simulink model "sm_aerial_trajectory"  (R2020b)
settings: Solver=ode45  StartTime=0.0  StopTime=2*T_gait-T_stance  MaxStep=0.001  RelTol=1e-3  EnableMultiTasking=on
InitFcn:
  | if (~exist('T_gait') || ~exist('T_stance'))
  |   sm_robot_run_4legs_param_def_load(bdroot)
  | end
values from neighbouring files (symbols this model uses):
  accel_aerial = (-leg_angle0-(T_gait-T_stance/2)*leg_vel0)/(0.5*(T_gait-T_stance/2)^2)    [kinematic_walking.m]
  T_gait = leg_angle.time(end)    [kinematic_walking.m]
  T_stance = 2*stance.time(idx_stance)    [kinematic_walking.m]
undefined symbols (not defined in the file or in its folder): leg_angle0, leg_vel0
CloseFcn:
  | try,close(h1_sm_robot_run_02_aerial_trajectory),end
  | clear h1_sm_robot_run_02_aerial_trajectory
  | 
  | clear logsout_sm_robot_run_02_aerial_trajectory
Description:
  | Copyright 2012-2020 The MathWorks, Inc.
settings Model: Creator=rhyde  LastModifiedBy=tedsa
settings DataIOCC: SaveFormat=Array  ReturnWorkspaceOutputs=off  SignalLoggingName=logsout_sm_robot_run_02_aerial_trajectory
settings OptimizationCC: ExpressionDepthLimit=2147483647  InitFltsAndDblsToZero=on  LifeSpan=inf
settings DebuggingCC: UnderspecifiedInitializationDetection=Classic  MergeDetectMultiDrivingBlocksExec=none  SolverPrmCheckMsg=warning  FcnCallInpInsideContextMsg=warning  StateNameClashWarn=warning  PregeneratedLibrarySubsystemCodeDiagnostic=none  SFUnexpectedBacktrackingDiag=warning  SFNoUnconditionalDefaultTransitionDiag=warning  SFExecutionAtInitializationDiag=none  ArithmeticOperatorsInVariantConditions=warning
settings HardwareCC: ProdBitPerPointer=32  ProdBitPerSizeT=32  ProdBitPerPtrDiffT=32  ProdLargestAtomicFloat=None  ProdIntDivRoundTo=Undefined  ProdEndianess=Unspecified  ProdWordSize=32  ProdHWDeviceType=32-bit Generic
settings ModelReferenceCC: PropagateSignalLabelsOutOfModel=off
settings SFSimCC: SimUseLocalCustomCode=off  CustomCodeUndefinedFunction=UseInterfaceOnly
settings RTWCC: RTWUseLocalCustomCode=off
settings CodeAppCC: StateflowObjectComments=on
settings GRTTargetCC: TargetLangStandard=C89/C90 (ANSI)  CombineOutputUpdateFcns=off  GRTInterface=on
settings ConfigComp: CovMetricSettings=dw  CovSaveCumulativeToWorkspaceVar=on  CovSaveSingleToWorkspaceVar=on  CovExternalEMLEnable=off

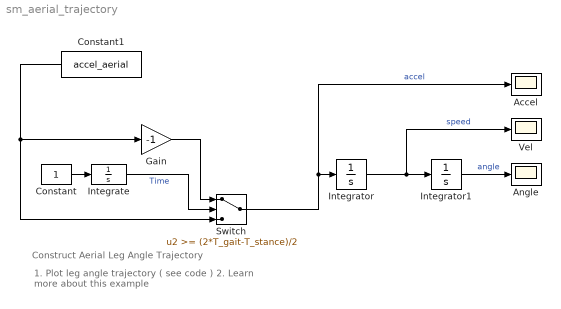
== system sm_aerial_trajectory ==
  note: Construct Aerial Leg Angle Trajectory
  note: 1. Plot leg angle trajectory ( see code )
      | 2. Learn more about this example
  Accel : Scope
  Angle : Scope
  Constant : Constant
  Constant1 : Constant  Value=accel_aerial
  Gain : Gain  Gain=-1
  Integrate : Integrator
  Integrator : Integrator  InitialCondition=leg_vel0
      settings: AttributesFormatString=%<InitialCondition>
  Integrator1 : Integrator  InitialCondition=leg_angle0
      settings: AttributesFormatString=%<InitialCondition>
  Switch : Switch  Threshold=(2*T_gait-T_stance)/2
      settings: AttributesFormatString=Threshold = %<Threshold>
  Vel : Scope
  wires:
  Integrate/1 -> Switch/2  "Time"
  Constant1/1 -> Switch/3, Gain/1
  Gain/1 -> Switch/1
  Switch/1 -> Integrator/1, Accel/1  "accel"
  Integrator/1 -> Integrator1/1, Vel/1  "speed"
  Integrator1/1 -> Angle/1  "angle"
  Constant/1 -> Integrate/1
